simulink model "PositionComplementary4"  (Simulink 6.6)
settings: Solver=ode4  StartTime=0.0  StopTime=inf  FixedStep=SampleT  RelTol=1e-3
InitFcn:
  | clc
  | Taxi_Var_new
  | failures
  | insInit
  | piccolo_init
values from neighbouring files (symbols this model uses):
  A1 = 0    [Taxi_Var.m]    (also in Taxi_Var_new.m = 0.007)
  Apolar = 0.0899    [Taxi_Var.m]    (also in Taxi_Var_new.m = 0.057)
  CD0 = 0.0219    [Taxi_Var.m]    (also in Taxi_Var_new.m = 0.022)
  chord = S/span    (= 0.384036716878)    [Taxi_Var.m]    (also in Taxi_Var_new.m = 0.351341681574)
  CL0 = 0.1857    [Taxi_Var.m]    (also in Taxi_Var_new.m = 0.38)
  CLa = 4.6206    [Taxi_Var.m]    (also in Taxi_Var_new.m = 18.5)
  CLa_dot = 1.93    [Taxi_Var.m]    (also in Taxi_Var_new.m = 2.64)
  Clb = -0.0043    [Taxi_Var.m]    (also in Taxi_Var_new.m = -0.06)
  ClDa = 0.1695    [Taxi_Var.m]    (also in Taxi_Var_new.m)
  CLDe = 0.4032    [Taxi_Var.m]    (also in Taxi_Var_new.m = 0.24)
  CLDf = 0.047    [Taxi_Var.m]    (also in Taxi_Var_new.m = 0.4)
  ClDr = 0.0003    [Taxi_Var.m]    (also in Taxi_Var_new.m = 0.055)
  Clp = -0.4425    [Taxi_Var.m]    (also in Taxi_Var_new.m = -0.88)
  CLq = 8.7465    [Taxi_Var.m]    (also in Taxi_Var_new.m = 7.4)
  Clr = 0.0675    [Taxi_Var.m]    (also in Taxi_Var_new.m = 0.04)
  Cm0 = -0.0902    [Taxi_Var.m]    (also in Taxi_Var_new.m = 0.56)
  Cma = -1.3995    [Taxi_Var.m]    (also in Taxi_Var_new.m = -1.58)
  CmDe = -0.9493    [Taxi_Var.m]    (also in Taxi_Var_new.m = -41)
  CmDf = -.021    (= -0.021)    [Taxi_Var.m]    (also in Taxi_Var_new.m)
  Cmq = -10.8760    (= -10.876)    [Taxi_Var.m]    (also in Taxi_Var_new.m = -12)
  Cnb = 0.0281    [Taxi_Var.m]    (also in Taxi_Var_new.m = 0.73)
  CnDa = -0.0031    [Taxi_Var.m]    (also in Taxi_Var_new.m = -0.032)
  CnDr = -0.0882    [Taxi_Var.m]    (also in Taxi_Var_new.m = 0.19)
  Cnp = -0.0695    [Taxi_Var.m]    (also in Taxi_Var_new.m = -0.1)
  Cnr = -0.1045    [Taxi_Var.m]    (also in Taxi_Var_new.m = -0.23)
  CYb = -0.1999    [Taxi_Var.m]    (also in Taxi_Var_new.m = -0.98)
  CYDr = 0.0192    [Taxi_Var.m]    (also in Taxi_Var_new.m = 0.066)
  damax = 25*deg2rad    (= 0.436332312999)    [Taxi_Var.m]    (also in piccolo_init.m)
  damin = -25*deg2rad    (= -0.436332312999)    [Taxi_Var.m]    (also in piccolo_init.m)
  datrim = 0*deg2rad    (= 0)    [Taxi_Var.m]    (also in piccolo_init.m)
  demax = 15*deg2rad    (= 0.261799387799)    [Taxi_Var.m]    (also in piccolo_init.m)
  demin = -15*deg2rad    (= -0.261799387799)    [Taxi_Var.m]    (also in piccolo_init.m)
  detrim = -2.4137*deg2rad    (= -0.0421270121554)    [Taxi_Var.m]    (also in piccolo_init.m = -0.0523598775598)
  dfland = 30*deg2rad    (= 0.523598775598)    [Taxi_Var.m]    (also in piccolo_init.m)
  dfmax = 30*deg2rad    (= 0.523598775598)    [Taxi_Var.m]    (also in piccolo_init.m)
  dfmin = 0*deg2rad    (= 0)    [Taxi_Var.m]    (also in piccolo_init.m)
  drmax = 25*deg2rad    (= 0.436332312999)    [Taxi_Var.m]    (also in piccolo_init.m)
  drmin = -25*deg2rad    (= -0.436332312999)    [Taxi_Var.m]    (also in piccolo_init.m)
  drtrim = 0*deg2rad    (= 0)    [Taxi_Var.m]    (also in piccolo_init.m)
  dtmax = 1    [Taxi_Var.m]    (also in piccolo_init.m = 0.7)
  dtmin = 0    [Taxi_Var.m]    (also in piccolo_init.m = 0.25)
  dttrim = 0.0725    [Taxi_Var.m]    (also in piccolo_init.m = 0.35)
  Euler_0 = [0; 0; 45]'*pi/180    [Taxi_Var.m]    (also in Taxi_Var_new.m = [0 0 45]'*pi/180)
  IdxCmdOrbitRadius = 17    [piccolo_init.m]
  IdxCmdOrbitSense = 18    [piccolo_init.m]
  IdxCmdWp1Alt = 13    [piccolo_init.m]
  IdxCmdWp1Lat = 11    [piccolo_init.m]
  IdxCmdWp1Lon = 12    [piccolo_init.m]
  IdxCmdWp2Alt = 16    [piccolo_init.m]
  IdxCmdWp2Lat = 14    [piccolo_init.m]
  IdxCmdWp2Lon = 15    [piccolo_init.m]
  IdxEstimReserved1 = 4    [piccolo_init.m]
  IdxEstimWEast = 3    [piccolo_init.m]
  IdxEstimWNorth = 2    [piccolo_init.m]
  IdxGainsAltD = 10    [piccolo_init.m]
  IdxGainsAltI = 9    [piccolo_init.m]
  IdxGainsAltP = 8    [piccolo_init.m]
  IdxGainsPdynD = 4    [piccolo_init.m]
  IdxGainsPdynI = 3    [piccolo_init.m]
  IdxGainsPdynP = 2    [piccolo_init.m]
  IdxGainsPitchD = 7    [piccolo_init.m]
  IdxGainsPitchI = 6    [piccolo_init.m]
  IdxGainsPitchP = 5    [piccolo_init.m]
  IdxGainsRollD = 17    [piccolo_init.m]
  IdxGainsRollI = 16    [piccolo_init.m]
  IdxGainsRollP = 15    [piccolo_init.m]
  IdxGainsSlopeElevatorD = 25    [piccolo_init.m]
  IdxGainsSlopeElevatorP = 26    [piccolo_init.m]
  IdxGainsTrackConv = 24    [piccolo_init.m]
  IdxGainsTrackD = 23    [piccolo_init.m]
  IdxGainsTrackI = 22    [piccolo_init.m]
  IdxGainsTrackP = 21    [piccolo_init.m]
  IdxGainsTurnD = 14    [piccolo_init.m]
  IdxGainsTurnI = 13    [piccolo_init.m]
  IdxGainsTurnP = 12    [piccolo_init.m]
  IdxGainsYawD = 20    [piccolo_init.m]
  IdxGainsYawI = 19    [piccolo_init.m]
  IdxGainsYawP = 18    [piccolo_init.m]
  IdxLimitsAileronMax = 11    [piccolo_init.m]
  IdxLimitsAileronMin = 10    [piccolo_init.m]
  IdxLimitsBankMax = 9    [piccolo_init.m]
  IdxLimitsBankMin = 8    [piccolo_init.m]
  IdxLimitsElevatorMax = 13    [piccolo_init.m]
  IdxLimitsElevatorMin = 12    [piccolo_init.m]
  IdxLimitsFlapMax = 19    [piccolo_init.m]
  IdxLimitsFlapMin = 18    [piccolo_init.m]
  IdxLimitsPdynMax = 3    [piccolo_init.m]
  IdxLimitsPdynMin = 2    [piccolo_init.m]
  IdxLimitsRudderMax = 15    [piccolo_init.m]
  IdxLimitsRudderMin = 14    [piccolo_init.m]
  IdxLimitsThrottleMax = 17    [piccolo_init.m]
  IdxLimitsThrottleMin = 16    [piccolo_init.m]
  IdxSensorsAlt = 5    [piccolo_init.m]
  IdxSensorsLat = 3    [piccolo_init.m]
  IdxSensorsLon = 4    [piccolo_init.m]
  IdxSensorsVDown = 8    [piccolo_init.m]
  IdxSensorsVEast = 7    [piccolo_init.m]
  IdxSensorsVNorth = 6    [piccolo_init.m]
  IdxStatesGlobal = 2    [piccolo_init.m]
  IdxStatesManual = 16    [piccolo_init.m]
  IdxStatesMode = 15    [piccolo_init.m]
  ISA_g = 9.815    [Taxi_Var.m]    (also in Taxi_Var_new.m)
  ISA_hmax = 2000    [Taxi_Var.m]    (also in Taxi_Var_new.m)
  ISA_lapse = .0065    (= 0.0065)    [Taxi_Var.m]    (also in Taxi_Var_new.m)
  ISA_P0 = 101325    [Taxi_Var.m]    (also in Taxi_Var_new.m)
  ISA_R = 287    [Taxi_Var.m]    (also in Taxi_Var_new.m)
  ISA_rho0 = 1.225    [Taxi_Var.m]    (also in Taxi_Var_new.m)
  ISA_T0 = 289    [Taxi_Var.m]    (also in Taxi_Var_new.m)
  Ixx = 3.689084    [Taxi_Var.m]    (also in Taxi_Var_new.m = 3.8)
  Iyy = 7.43789    [Taxi_Var.m]    (also in Taxi_Var_new.m = 9.58)
  Izz = 10.22202    [Taxi_Var.m]    (also in Taxi_Var_new.m = 9.68)
  mass = 22.5    [Taxi_Var.m]    (also in Taxi_Var_new.m = 8.16466266)
  MinThK = 0.075    [Taxi_Var.m]    (also in Taxi_Var_new.m = 0.077)
  Pos_0 = [0; 0; 1000]'    [Taxi_Var.m]    (also in Taxi_Var_new.m = [0 0 500]')
  PQR_0 = [0; 0; 0]'    [Taxi_Var.m]    (also in Taxi_Var_new.m = [ 0 0 0]'*pi/180)
  SampleT = 0.005    [failures.m]
  span = 2.3368    [Taxi_Var.m]    (also in Taxi_Var_new.m = 2.795)
  TFact = 0.4    [Taxi_Var.m]    (also in Taxi_Var_new.m)
  ThK = 2.18    [Taxi_Var.m]    (also in Taxi_Var_new.m = 2.17)
  tsamp = APtsamp    (= 0.05)    [piccolo_init.m]
  ... (+1 more)
undefined symbols (not defined in the file or in its folder): clock, DiscIntNeverNeededParam, Earth, gaind, polesd, WGS84, zerosd
libraries: piccolo_library x60, simulink x55, aerolibconvert2 x18, aerolibasang x5, dspsigops x5, aerolibtransform2 x2, aerolibatmos2 x2, aerolibnav x2, aerolibguid x1, aerolibutil x1, dspmtrx3 x1
(part 2 of 7)

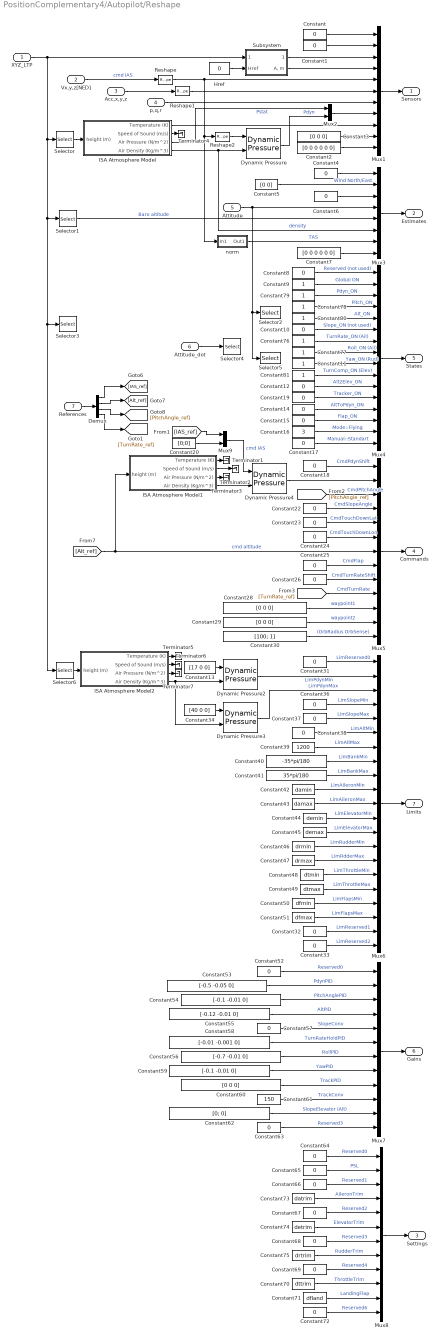
== system PositionComplementary4/Autopilot/Reshape ==
  XYZ_LTP : Inport  OutDataType=fixdt(1,16,0)  OutScaling=[]
  Vx,y,z[NED] : Inport  Port=2  OutDataType=fixdt(1,16,0)  OutScaling=[]
  Acc,x,y,z : Inport  Port=3  OutDataType=fixdt(1,16,0)  OutScaling=[]
  p,q,r : Inport  Port=4  OutDataType=fixdt(1,16,0)  OutScaling=[]
  Attitude : Inport  Port=5  OutDataType=fixdt(1,16,0)  OutScaling=[]
  Attitude_dot : Inport  Port=6  OutDataType=fixdt(1,16,0)  OutScaling=[]
  References : Inport  Port=7  OutDataType=fixdt(1,16,0)  OutScaling=[]
  Constant{,1,4,6,8,10,12,14..15,17..19,22..26,31..33,36..38,52,57,63..69,72} (33 alike) : Constant  Value=0
  Constant{9,11,76..81} (8 alike) : Constant
  Constant13 : Constant  Value=[17 0 0]
  Constant16 : Constant  Value=3
  Constant2 : Constant  Value=[0 0 0 0 0 0]
  Constant20 : Constant  Value=[0;0]
  Constant{3,28..29,60} (4 alike) : Constant  Value=[0 0 0]
  Constant30 : Constant  Value=[100; 1]
  Constant34 : Constant  Value=[40 0 0]
  Constant39 : Constant  Value=1200
  Constant40 : Constant  Value=-35*pi/180
  Constant41 : Constant  Value=35*pi/180
  Constant42 : Constant  Value=damin
  Constant43 : Constant  Value=damax
  Constant44 : Constant  Value=demin
  Constant45 : Constant  Value=demax
  Constant46 : Constant  Value=drmin
  Constant47 : Constant  Value=drmax
  Constant48 : Constant  Value=dtmin
  Constant49 : Constant  Value=dtmax
  Constant5 : Constant  Value=[0 0]
  Constant50 : Constant  Value=dfmin
  Constant51 : Constant  Value=dfmax
  Constant53 : Constant  Value=[-0.5 -0.05 0]
  Constant54 : Constant  Value=[-0.1 -0.01 0]
  Constant55 : Constant  Value=[-0.12 -0.01 0]
  Constant56 : Constant  Value=[-0.7 -0.01 0]
  Constant58 : Constant  Value=[-0.01 -0.001 0]
  Constant59 : Constant  Value=[-0.1 -0.01 0]
  Constant61 : Constant  Value=150
  Constant62 : Constant  Value=[0; 0]
  Constant7 : Constant  Value=[0 0 0 0 0 0]
  Constant70 : Constant  Value=dttrim
  Constant71 : Constant  Value=dfland
  Constant73 : Constant  Value=datrim
  Constant74 : Constant  Value=detrim
  Constant75 : Constant  Value=drtrim
  Demux : Demux
  Dynamic Pressure{,2..4} (4 alike) : aerolibasang/Dynamic Pressure  SystemSampleTime=-1
  Href : Constant  Value=0
  ISA Atmosphere Model : Subsystem  mask(International Standart Atmosphere){L=ISA_lapse, h_lim=ISA_hmax, R=ISA_R, g=ISA_g, rh0=ISA_rho0, P0=ISA_P0, T0=ISA_T0}
      mask prompts: L "Lapse rate"; h_lim "Upper altitude limit, (m)"; R "Universal gas constant R"; g "Garvity constant, (m/c^2)"; rh0 "Sea level density, (kg/m^3)"; P0 "Sea level pressure, (N/m^2)"; T0 "Sea level temperature, (K)"
  ISA Atmosphere Model1 : Subsystem  mask(International Standart Atmosphere){L=ISA_lapse, h_lim=ISA_hmax, R=ISA_R, g=ISA_g, rh0=ISA_rho0, P0=ISA_P0, T0=ISA_T0}
      mask prompts: L "Lapse rate"; h_lim "Upper altitude limit, (m)"; R "Universal gas constant R"; g "Garvity constant, (m/c^2)"; rh0 "Sea level density, (kg/m^3)"; P0 "Sea level pressure, (N/m^2)"; T0 "Sea level temperature, (K)"
  ISA Atmosphere Model2 : Subsystem  mask(International Standart Atmosphere){L=ISA_lapse, h_lim=ISA_hmax, R=ISA_R, g=ISA_g, rh0=ISA_rho0, P0=ISA_P0, T0=ISA_T0}
      mask prompts: L "Lapse rate"; h_lim "Upper altitude limit, (m)"; R "Universal gas constant R"; g "Garvity constant, (m/c^2)"; rh0 "Sea level density, (kg/m^3)"; P0 "Sea level pressure, (N/m^2)"; T0 "Sea level temperature, (K)"
  Mux1 : Mux  Inputs=11
  Mux2 : Mux  Inputs=2
  Mux3 : Mux  Inputs=8
  Mux4 : Mux  Inputs=16
  Mux5 : Mux  Inputs=13
  Mux6 : Mux  Inputs=21
  Mux7 : Mux  Inputs=12
  Mux8 : Mux  Inputs=12
  Mux9 : Mux  Inputs=2
  Reshape : Reshape
  Reshape1 : Reshape
  Reshape2 : Reshape
  Selector{,1,3..4,6} (5 alike) : Selector  IndexOptions=Index vector (dialog)  Indices=3  OutputSizes=[(-2)]  InputPortWidth=3
  Selector2 : Selector  IndexOptions=Index vector (dialog)  Indices=2  OutputSizes=[(-2)]  InputPortWidth=3
  Selector5 : Selector  IndexOptions=Index vector (dialog)  Indices=[1 3]  OutputSizes=[(-2)]  InputPortWidth=3
  Subsystem : Subsystem
  Terminator{1..7} (7 alike) : Terminator
  norm : Subsystem
  Sensors : Outport  OutDataType=fixdt(1,16,0)  OutScaling=[]
  Estimates : Outport  Port=2  OutDataType=fixdt(1,16,0)  OutScaling=[]
  Settings : Outport  Port=3  OutDataType=fixdt(1,16,0)  OutScaling=[]
  Commands : Outport  Port=4  OutDataType=fixdt(1,16,0)  OutScaling=[]
  States : Outport  Port=5  OutDataType=fixdt(1,16,0)  OutScaling=[]
  Gains : Outport  Port=6  OutDataType=fixdt(1,16,0)  OutScaling=[]
  Limits : Outport  Port=7  OutDataType=fixdt(1,16,0)  OutScaling=[]
  wires:
  Constant/1 -> Mux1/1
  Constant1/1 -> Mux1/2
  Subsystem/1("LL, deg") -> Mux1/3
  Subsystem/2("A, m") -> Mux1/4
  XYZ_LTP/1 -> Subsystem/1("XYZ, ltp"), Selector/1, Selector1/1, Selector3/1, Selector6/1
  Vx,y,z[NED]/1 -> Reshape/1  "cmd IAS"
  Mux1/1 -> Sensors/1
  Acc,x,y,z/1 -> Reshape1/1
  p,q,r/1 -> Mux1/7
  Constant3/1 -> Mux1/10
  Constant2/1 -> Mux1/11
  ISA Atmosphere Model/4(Air Density (Kg/m^3)) -> Dynamic Pressure/2, Mux3/6  "density"
  ISA Atmosphere Model/1(Temperature (K)) -> Mux1/9
  Mux2/1 -> Mux1/8
  ISA Atmosphere Model/3("Air Pressure (N/m^2) ") -> Mux2/1  "Pstat"
  ISA Atmosphere Model/2("Speed of Sound (m/s) ") -> Terminator4/1
  Dynamic Pressure/1 -> Mux2/2  "Pdyn"
  Selector/1 -> ISA Atmosphere Model/1(height (m))
  Reshape/1 -> Mux1/5, Reshape2/1, norm/1(In1)
  Reshape1/1 -> Mux1/6
  Reshape2/1 -> Dynamic Pressure/1
  Href/1 -> Subsystem/2(Href)
  Mux3/1 -> Estimates/1
  Constant4/1 -> Mux3/1
  Constant5/1 -> Mux3/2  "Wind North/East"
  Constant6/1 -> Mux3/3
  Attitude/1 -> Selector2/1, Selector5/1, Mux3/4
  Selector1/1 -> Mux3/5  "Baro altitude"
  norm/1(Out1) -> Mux3/7  "TAS"
  Constant7/1 -> Mux3/8
  Mux4/1 -> States/1
  Constant8/1 -> Mux4/1  "Reserved (not used)"
  Constant9/1 -> Mux4/2  "Global ON"
  Constant10/1 -> Mux4/6  "Slope_ON (not used)"
  Attitude_dot/1 -> Selector4/1
  Constant11/1 -> Mux4/9  "Yaw_ON (Rud)"
  Mux5/1 -> Commands/1
  Constant18/1 -> Mux5/1  "CmdPdynShift"
  ISA Atmosphere Model1/1(Temperature (K)) -> Terminator1/1
  ISA Atmosphere Model1/2("Speed of Sound (m/s) ") -> Terminator2/1
  ISA Atmosphere Model1/3("Air Pressure (N/m^2) ") -> Terminator3/1
  ISA Atmosphere Model1/4(Air Density (Kg/m^3)) -> Dynamic Pressure4/2
  Dynamic Pressure4/1 -> Mux5/2
  Mux9/1 -> Dynamic Pressure4/1  "cmd IAS"
  [Alt_ref] -> ISA Atmosphere Model1/1(height (m)), Mux5/7  "cmd altitude"
  [PitchAngle_ref] -> Mux5/3  "CmdPitchAngle"
  Constant22/1 -> Mux5/4  "CmdSlopeAngle"
  Constant24/1 -> Mux5/6  "CmdTouchDownLon"
  Constant23/1 -> Mux5/5  "CmdTouchDownLat"
  Constant25/1 -> Mux5/8  "CmdFlap"
  Constant26/1 -> Mux5/9  "CmdTurnRateShift"
  [TurnRate_ref] -> Mux5/10  "CmdTurnRate"
  Constant28/1 -> Mux5/11  "waypoint1"
  Constant29/1 -> Mux5/12  "waypoint2"
  Constant30/1 -> Mux5/13  "(OrbRadius OrbSense)"
  Mux6/1 -> Limits/1
  Constant31/1 -> Mux6/1  "LimReserved0"
  Constant33/1 -> Mux6/21  "LimReserved2"
  Constant32/1 -> Mux6/20  "LimReserved1"
  ISA Atmosphere Model2/1(Temperature (K)) -> Terminator5/1
  ISA Atmosphere Model2/2("Speed of Sound (m/s) ") -> Terminator6/1
  ISA Atmosphere Model2/3("Air Pressure (N/m^2) ") -> Terminator7/1
  ISA Atmosphere Model2/4(Air Density (Kg/m^3)) -> Dynamic Pressure2/2, Dynamic Pressure3/2
  Constant13/1 -> Dynamic Pressure2/1
  Constant34/1 -> Dynamic Pressure3/1
  Selector6/1 -> ISA Atmosphere Model2/1(height (m))
  Dynamic Pressure2/1 -> Mux6/2  "LimPdynMin"
  Dynamic Pressure3/1 -> Mux6/3  "LimPdynMax"
  Constant36/1 -> Mux6/4  "LimSlopeMin"
  Constant37/1 -> Mux6/5  "LimSlopeMax"
  Constant38/1 -> Mux6/6  "LimAltMin"
  Constant39/1 -> Mux6/7  "LimAltMax"
  Constant40/1 -> Mux6/8  "LimBankMin"
  Constant41/1 -> Mux6/9  "LimBankMax"
  Constant42/1 -> Mux6/10  "LimAileronMin"
  Constant43/1 -> Mux6/11  "LimAileronMax"
  Constant44/1 -> Mux6/12  "LimElevatorMin"
  Constant45/1 -> Mux6/13  "LimElevatorMax"
  Constant46/1 -> Mux6/14  "LimRudderMin"
  Constant47/1 -> Mux6/15  "LimRdderMax"
  Constant48/1 -> Mux6/16  "LimThrottleMin"
  Constant49/1 -> Mux6/17  "LimThrottleMax"
  Constant50/1 -> Mux6/18  "LimFlapsMin"
  Constant51/1 -> Mux6/19  "LimFlapsMax"
  Mux7/1 -> Gains/1
  Constant52/1 -> Mux7/1  "Reserved0"
  Constant53/1 -> Mux7/2  "PdynPID"
  Constant54/1 -> Mux7/3  "PitchAnglePID"
  Constant55/1 -> Mux7/4  "AltPID"
  Constant58/1 -> Mux7/6  "TurnRateHoldPID"
  Constant57/1 -> Mux7/5  "SlopeConv"
  Constant56/1 -> Mux7/7  "RollPID"
  Constant59/1 -> Mux7/8  "YawPID"
  Constant60/1 -> Mux7/9  "TrackPID"
  Constant61/1 -> Mux7/10  "TrackConv"
  Constant62/1 -> Mux7/11  "SlopeElevator (Alt)"
  Constant63/1 -> Mux7/12  "Reserved3"
  Mux8/1 -> Settings/1
  Constant64/1 -> Mux8/1  "Reserved0"
  Constant65/1 -> Mux8/2  "PSL"
  Constant66/1 -> Mux8/3  "Reserved1"
  Constant67/1 -> Mux8/5  "Reserved2"
  Constant68/1 -> Mux8/7  "Reserved3"
  Constant69/1 -> Mux8/9  "Reserved4"
  Constant70/1 -> Mux8/10  "ThrottleTrim"
  Constant71/1 -> Mux8/11  "LandingFlap"
  Constant72/1 -> Mux8/12  "Reserved6"
  Constant73/1 -> Mux8/4  "AileronTrim"
  Constant74/1 -> Mux8/6  "ElevatorTrim"
  Constant75/1 -> Mux8/8  "RudderTrim"
  Constant76/1 -> Mux4/7  "TurnRate_ON (Ail)"
  Constant77/1 -> Mux4/8  "Roll_ON (Ail)"
  Constant78/1 -> Mux4/4  "Pitch_ON"
  Constant79/1 -> Mux4/3  "Pdyn_ON"
  Constant80/1 -> Mux4/5  "Alt_ON"
  Constant81/1 -> Mux4/10  "TurnComp_ON (Elev)"
  Constant12/1 -> Mux4/11  "Alt2Elev_ON"
  Constant19/1 -> Mux4/12  "Tracker_ON"
  Constant14/1 -> Mux4/13  "AltToPdyn_ON"
  Constant15/1 -> Mux4/14  "Flap_ON"
  Constant16/1 -> Mux4/15  "Mode::Flying"
  Constant17/1 -> Mux4/16  "Manual::Standart"
  References/1 -> Demux/1
  Demux/1 -> [IAS_ref]
  Demux/2 -> [Alt_ref]
  Demux/3 -> [PitchAngle_ref]
  Demux/4 -> [TurnRate_ref]
  Constant20/1 -> Mux9/2
  [IAS_ref] -> Mux9/1

== system PositionComplementary4/GPS Update/Detect Change ==
  Data : Inport
  Abs1 : Abs  SampleTime=T
  Difference1 : simulink/Discrete/Difference  SystemSampleTime=-1  ICPrevInput=0.0  OutDataType=sfix(16)  OutScaling=2^-10  DoSatur=off
  Saturation1 : Saturate  UpperLimit=1  LowerLimit=0  SampleTime=T
  change? : Outport
  wires:
  Difference1/1 -> Abs1/1
  Abs1/1 -> Saturation1/1
  Data/1 -> Difference1/1
  Saturation1/1 -> change?/1

== system PositionComplementary4/GPS Update/Detect Change1 ==
  Data : Inport
  Abs1 : Abs  SampleTime=T
  Difference1 : simulink/Discrete/Difference  SystemSampleTime=-1  ICPrevInput=0.0  OutDataType=sfix(16)  OutScaling=2^-10  DoSatur=off
  Saturation1 : Saturate  UpperLimit=1  LowerLimit=0  SampleTime=T
  change? : Outport
  wires:
  Saturation1/1 -> change?/1
  Data/1 -> Difference1/1
  Abs1/1 -> Saturation1/1
  Difference1/1 -> Abs1/1

== system PositionComplementary4/GPS Update/Detect Change2 ==
  Data : Inport
  Abs1 : Abs  SampleTime=T
  Difference1 : simulink/Discrete/Difference  SystemSampleTime=-1  ICPrevInput=0.0  OutDataType=sfix(16)  OutScaling=2^-10  DoSatur=off
  Saturation1 : Saturate  UpperLimit=1  LowerLimit=0  SampleTime=T
  change? : Outport
  wires:
  Difference1/1 -> Abs1/1
  Abs1/1 -> Saturation1/1
  Data/1 -> Difference1/1
  Saturation1/1 -> change?/1

== system PositionComplementary4/Get GPS in LTP/Geod2LTP2 ==
  "Height, Lat, Lon Initials from GPS" : Inport
  "Lat, deg(GPS)" : Inport  Port=2
  "Lon, deg(GPS)" : Inport  Port=3
  Hight,m(GPS) : Inport  Port=4
  Demux : Demux  Outputs=3
  ECEF2LTP (UEN) : Subsystem
      mask Display: plot(0,0,100,100,[45,40,35,40,40],[85,95,85,95,40],[85,95,85,95,40],[35,40,45,40,40],[60,40,10,20,10,14],[70,40,10,13,10,20],[56,45],[70,70],[60,60],[50,60],[60,60],[30,40],[50,60],[20,20],[30,40],[20,20],[45,55],[35,25],[75,65],[35,25])
  Geod2ECEF : Subsystem  mask{Re=6378137, Rp=6356752.3142}
      mask prompts: Re "Enter equatorial radius, m"; Rp "Enter polar radius,m"
  Geod2ECEF1 : Subsystem  mask{Re=6378137, Rp=6356752.3142}
      mask prompts: Re "Enter equatorial radius, m"; Rp "Enter polar radius,m"
  Mux : Mux  Inputs=3
  Mux1 : Mux  Inputs=2
  Mux2 : Mux  Inputs=3
  Reshape : Reshape  OutputDimensionality=Column vector (2-D)
  Sum1 : Sum  Inputs=|+-  SaturateOnIntegerOverflow=on
  UEN 2 NEU : Gain  Gain=[0 0 1;0 1 0;1 0 0]  Multiplication=Matrix(K*u)  SaturateOnIntegerOverflow=on
  "NEU, m" : Outport
  wires:
  UEN 2 NEU/1 -> "NEU, m"/1
  Geod2ECEF/3("Ze, m ") -> Mux/3
  Geod2ECEF/1("Xe, m ") -> Mux/1
  Geod2ECEF/2("Ye, m ") -> Mux/2
  "Lat, deg(GPS)"/1 -> Geod2ECEF/2("lat, deg")
  "Lon, deg(GPS)"/1 -> Geod2ECEF/3(lon,deg)
  Mux1/1 -> ECEF2LTP (UEN)/2("Long, Lat")
  Geod2ECEF1/3("Ze, m ") -> Mux2/3
  Geod2ECEF1/1("Xe, m ") -> Mux2/1
  Geod2ECEF1/2("Ye, m ") -> Mux2/2
  Mux2/1 -> Sum1/2  "R_in"
  Demux/1 -> Geod2ECEF1/1("height, m")
  Demux/2 -> Mux1/2, Geod2ECEF1/2("lat, deg")
  Demux/3 -> Mux1/1, Geod2ECEF1/3(lon,deg)
  ECEF2LTP (UEN)/1(Out) -> Reshape/1  "Moving Side"
  Hight,m(GPS)/1 -> Geod2ECEF/1("height, m")
  "Height, Lat, Lon Initials from GPS"/1 -> Demux/1
  Mux/1 -> Sum1/1  "r_mov"
  Sum1/1 -> ECEF2LTP (UEN)/1(ECEF coordinates)
  Reshape/1 -> UEN 2 NEU/1

== system PositionComplementary4/Get GPS in LTP/Sim Latency ==
  Fast Data : Inport
  Data Type Conversion : DataTypeConversion  OutDataTypeMode=double
  Pulse Generator : DiscretePulseGenerator  PulseType=Time based  PulseWidth=50
  Rate Transition2 : RateTransition  OutPortSampleTime=SampleT
  Sample and Hold : dspsigops/Sample and Hold  SystemSampleTime=-1  trig=Either edge  initCond=0  latchinput=off
  1Hz Data : Outport
  wires:
  Data Type Conversion/1 -> Rate Transition2/1
  Sample and Hold/1 -> 1Hz Data/1
  Fast Data/1 -> Sample and Hold/1
  Rate Transition2/1 -> Sample and Hold/Trigger
  Pulse Generator/1 -> Data Type Conversion/1

== system PositionComplementary4/Get GPS in LTP/Sim Latency1 ==
  Fast Data : Inport
  Data Type Conversion : DataTypeConversion  OutDataTypeMode=double
  Pulse Generator : DiscretePulseGenerator  PulseType=Time based  PulseWidth=50
  Rate Transition2 : RateTransition  OutPortSampleTime=SampleT
  Sample and Hold : dspsigops/Sample and Hold  SystemSampleTime=-1  trig=Either edge  initCond=0  latchinput=off
  1Hz Data : Outport
  wires:
  Pulse Generator/1 -> Data Type Conversion/1
  Rate Transition2/1 -> Sample and Hold/Trigger
  Fast Data/1 -> Sample and Hold/1
  Sample and Hold/1 -> 1Hz Data/1
  Data Type Conversion/1 -> Rate Transition2/1

== system PositionComplementary4/Get GPS in LTP/Sim Latency2 ==
  Fast Data : Inport
  Data Type Conversion : DataTypeConversion  OutDataTypeMode=double
  Pulse Generator : DiscretePulseGenerator  PulseType=Time based  PulseWidth=50
  Rate Transition2 : RateTransition  OutPortSampleTime=SampleT
  Sample and Hold : dspsigops/Sample and Hold  SystemSampleTime=-1  trig=Either edge  initCond=0  latchinput=off
  1Hz Data : Outport
  wires:
  Data Type Conversion/1 -> Rate Transition2/1
  Sample and Hold/1 -> 1Hz Data/1
  Fast Data/1 -> Sample and Hold/1
  Rate Transition2/1 -> Sample and Hold/Trigger
  Pulse Generator/1 -> Data Type Conversion/1

== system PositionComplementary4/Get GPS in LTP/Sim Latency3 ==
  Fast Data : Inport
  Data Type Conversion : DataTypeConversion  OutDataTypeMode=double
  Pulse Generator : DiscretePulseGenerator  PulseType=Time based  PulseWidth=50
  Rate Transition2 : RateTransition  OutPortSampleTime=SampleT
  Sample and Hold : dspsigops/Sample and Hold  SystemSampleTime=-1  trig=Either edge  initCond=0  latchinput=off
  1Hz Data : Outport
  wires:
  Pulse Generator/1 -> Data Type Conversion/1
  Rate Transition2/1 -> Sample and Hold/Trigger
  Fast Data/1 -> Sample and Hold/1
  Sample and Hold/1 -> 1Hz Data/1
  Data Type Conversion/1 -> Rate Transition2/1

== system PositionComplementary4/Get GPS in LTP/Sim Latency4 ==
  Fast Data : Inport
  Data Type Conversion : DataTypeConversion  OutDataTypeMode=double
  Pulse Generator : DiscretePulseGenerator  PulseType=Time based  PulseWidth=50
  Rate Transition2 : RateTransition  OutPortSampleTime=SampleT
  Sample and Hold : dspsigops/Sample and Hold  SystemSampleTime=-1  trig=Either edge  initCond=0  latchinput=off
  1Hz Data : Outport
  wires:
  Data Type Conversion/1 -> Rate Transition2/1
  Sample and Hold/1 -> 1Hz Data/1
  Fast Data/1 -> Sample and Hold/1
  Rate Transition2/1 -> Sample and Hold/Trigger
  Pulse Generator/1 -> Data Type Conversion/1

== system PositionComplementary4/Plant Model/Plant ==
  de : Inport
  da : Inport  Port=2
  dr : Inport  Port=3
  dt : Inport  Port=4
  df : Inport  Port=5
  6-DOF EOM : Subsystem
  Engine Model : Subsystem
  Forces and Moments : Subsystem
  Get GPS : Subsystem
  ISA Atmosphere & Winds : Subsystem  Orientation=left
  Mux : Mux  Inputs=2
  Scope : Scope
      settings: YMin=0  YMax=5250
  Sum : Sum  Inputs=++|  SaturateOnIntegerOverflow=on
  Wrap Around PSI1 : Subsystem
  GPS Month : Outport
  GPS Day : Outport  Port=2
  GPS Year : Outport  Port=3
  GPS Hr : Outport  Port=4
  GPS Min : Outport  Port=5
  GPS Sec : Outport  Port=6
  GPS Frac Sec : Outport  Port=7
  GPS Lat (rad) : Outport  Port=8
  GPS Long (rad) : Outport  Port=9
  GPS H (m) : Outport  Port=10
  PQR : Outport  Port=11
  Ab : Outport  Port=12
  Dynamic : Outport  Port=13
  Static : Outport  Orientation=left  Port=14
  Euler : Outport  Port=15
  Vmag : Outport  Port=16
  RPM : Outport  Port=17
  Vned : Outport  Port=18
  aoa/betta,deg : Outport  Port=19
  Ab meas : Outport  Port=20
  Vb : Outport  Port=21
  Euler_dot : Outport  Port=22
  wires:
  Get GPS/1(GPS Month) -> GPS Month/1
  Get GPS/2(GPS Day) -> GPS Day/1
  Get GPS/3(GPS Year) -> GPS Year/1
  Get GPS/4(GPS Hr) -> GPS Hr/1
  Get GPS/5(GPS Min) -> GPS Min/1
  Get GPS/6(GPS Sec) -> GPS Sec/1
  Get GPS/7(GPS Frac Sec) -> GPS Frac Sec/1
  Get GPS/8(GPS Lat (rad)) -> GPS Lat (rad)/1
  Get GPS/9(GPS Long (rad)) -> GPS Long (rad)/1
  Get GPS/10(GPS H (m)) -> GPS H (m)/1
  6-DOF EOM/8(Ab meas) -> Ab meas/1
  Mux/1 -> 6-DOF EOM/1("[F,M]")
  6-DOF EOM/5(Euler_dot) -> Euler_dot/1
  6-DOF EOM/6(Vb) -> Vb/1
  Engine Model/1(RPM) -> RPM/1
  Engine Model/2(Thrust) -> Sum/1
  Forces and Moments/6(q) -> Dynamic/1
  ISA Atmosphere & Winds/3(AirPressure (Pa)) -> Static/1
  Forces and Moments/1(Airspeed) -> Engine Model/2(Vmag), Vmag/1
  ISA Atmosphere & Winds/2(Wind) -> Forces and Moments/1(Wind e)
  ISA Atmosphere & Winds/1(Rho) -> Forces and Moments/2(Rho)
  Forces and Moments/3(Moments) -> Mux/2
  Forces and Moments/2(Forces) -> Sum/2
  Sum/1 -> Mux/1
  Forces and Moments/4(Vb Corr) -> 6-DOF EOM/2(Vb Corr)
  6-DOF EOM/1(X,Y,Z (LTP)) -> ISA Atmosphere & Winds/1("X, Y, Z"), Get GPS/1(XYZ (NEU)), Scope/1  "position"
  6-DOF EOM/2("Vx, Vy, Vz") -> Vned/1, Forces and Moments/7("Vx, Vy, Vz ")  "velocity"
  6-DOF EOM/3(Euler) -> Forces and Moments/8(Euler), Wrap Around PSI1/1(Euler)  "Euler angles"
  6-DOF EOM/4("p, q, r") -> PQR/1, Forces and Moments/9(p,q,r)  "rates"
  6-DOF EOM/7(Ab) -> Ab/1
  Forces and Moments/5("aoa/betta, deg") -> aoa/betta,deg/1
  dt/1 -> Engine Model/1(dt)
  de/1 -> Forces and Moments/3("de, deg")
  da/1 -> Forces and Moments/4(da,deg)
  dr/1 -> Forces and Moments/5("dr, deg")
  df/1 -> Forces and Moments/6("df, deg")
  Wrap Around PSI1/1(Euler-Wrapped) -> Euler/1

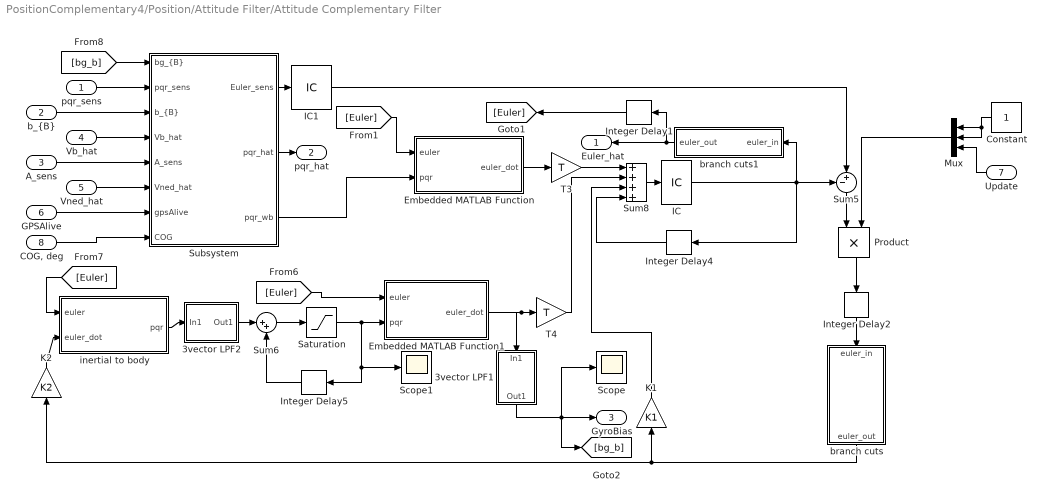
== system PositionComplementary4/Position/Attitude Filter/Attitude Complementary Filter ==
  pqr_sens : Inport
  "b_{B}" : Inport  Port=2
  A_sens : Inport  Port=3
  Vb_hat : Inport  Port=4
  Vned_hat : Inport  Port=5
  GPSAlive : Inport  Port=6
  Update : Inport  Orientation=left  Port=7
  "COG, deg" : Inport  Port=8
  3vector LPF1 : Subsystem  Orientation=down  mask{flpf=15, T=T}
      mask prompts: flpf "Low Pass Frequency (in S domain)"; T "Sample time"
      mask Display: droots([],-flpf,flpf)
  3vector LPF2 : Subsystem  mask{flpf=flpf, T=T}
      mask prompts: flpf "Low Pass Frequency (in S domain)"; T "Sample time"
      mask Display: droots([],-flpf,flpf)
  Constant : Constant  Orientation=left
  Embedded MATLAB Function : Stateflow chart
  Embedded MATLAB Function1 : Stateflow chart
  IC : InitialCondition  Value=P0  SampleTime=T
  IC1 : InitialCondition  Value=P0  SampleTime=T
  Integer Delay1 : simulink/Discrete/Integer Delay  Orientation=left  vinit=0.0  samptime=-1  NumDelays=1
  Integer Delay2 : simulink/Discrete/Integer Delay  Orientation=down  vinit=0.0  samptime=-1  NumDelays=1
  Integer Delay4 : simulink/Discrete/Integer Delay  Orientation=left  vinit=0.0  samptime=-1  NumDelays=1
  Integer Delay5 : simulink/Discrete/Integer Delay  Orientation=left  vinit=0.0  samptime=-1  NumDelays=1
  K1 : Gain  Orientation=up  Gain=K1
  K2 : Gain  Orientation=up  Gain=K2
  Mux : Mux  Orientation=left  Inputs=3
  Product : Product  Orientation=down  RndMeth=Zero
  Saturation : Saturate  UpperLimit=1.5  LowerLimit=-1.5
  Scope : Scope
      settings: TimeRange=60  YMin=-0.07116438310879042  YMax=0.01417979172834782  SaveName=ScopeData13
  Scope1 : Scope
      settings: TimeRange=60  YMin=-0.07116438310879042  YMax=0.01417979172834782  SaveName=ScopeData30
  Subsystem : Subsystem
  Sum5 : Sum  Orientation=down  Inputs=-+|
  Sum6 : Sum  Inputs=|++
  Sum8 : Sum  Inputs=4
  T3 : Gain  Gain=T  SampleTime=T
  T4 : Gain  Gain=T  SampleTime=T
  branch cuts : Stateflow chart  Orientation=down
  branch cuts1 : Stateflow chart  Orientation=left
  inertial to body : Stateflow chart
  Euler_hat : Outport  Orientation=left
  pqr_hat : Outport  Port=2
  GyroBias : Outport  Port=3
  wires:
  Embedded MATLAB Function/1(euler_dot) -> T3/1
  Subsystem/1(Euler_sens) -> IC1/1
  T3/1 -> Sum8/1
  Sum8/1 -> IC/1
  Integer Delay4/1 -> Sum8/4
  K1/1 -> Sum8/3
  inertial to body/1(pqr) -> 3vector LPF2/1(In1)
  Sum6/1 -> Saturation/1
  [Euler] -> Embedded MATLAB Function1/1(euler)
  [Euler] -> inertial to body/1(euler)
  Embedded MATLAB Function1/1(euler_dot) -> T4/1, 3vector LPF1/1(In1)
  T4/1 -> Sum8/2
  Integer Delay5/1 -> Sum6/2
  K2/1 -> inertial to body/2(euler_dot)
  [bg_b] -> Subsystem/1("bg_{B}")
  pqr_sens/1 -> Subsystem/2(pqr_sens)
  "b_{B}"/1 -> Subsystem/3("b_{B}")
  Vb_hat/1 -> Subsystem/4(Vb_hat)
  A_sens/1 -> Subsystem/5(A_sens)
  Vned_hat/1 -> Subsystem/6(Vned_hat)
  IC/1 -> Integer Delay4/1, Sum5/1, branch cuts1/1(euler_in)
  IC1/1 -> Sum5/2
  Integer Delay1/1 -> [Euler]
  [Euler] -> Embedded MATLAB Function/1(euler)
  Integer Delay2/1 -> branch cuts/1(euler_in)
  Subsystem/3(pqr_wb) -> Embedded MATLAB Function/2(pqr)
  Subsystem/2(pqr_hat) -> pqr_hat/1
  branch cuts/1(euler_out) -> K2/1, K1/1
  branch cuts1/1(euler_out) -> Euler_hat/1, Integer Delay1/1
  GPSAlive/1 -> Subsystem/7(gpsAlive)
  Product/1 -> Integer Delay2/1
  Sum5/1 -> Product/1
  "COG, deg"/1 -> Subsystem/8(COG)
  Constant/1 -> Mux/1, Mux/2
  Update/1 -> Mux/3
  Mux/1 -> Product/2
  3vector LPF2/1(Out1) -> Sum6/1
  3vector LPF1/1(Out1) -> GyroBias/1, [bg_b], Scope/1
  Saturation/1 -> Embedded MATLAB Function1/2(pqr), Integer Delay5/1, Scope1/1

== system PositionComplementary4/Position/Attitude Filter/Enabled Subsystem ==
  In1 : Inport
  Enable : EnablePort
  Out1 : Outport
  wires:
  In1/1 -> Out1/1

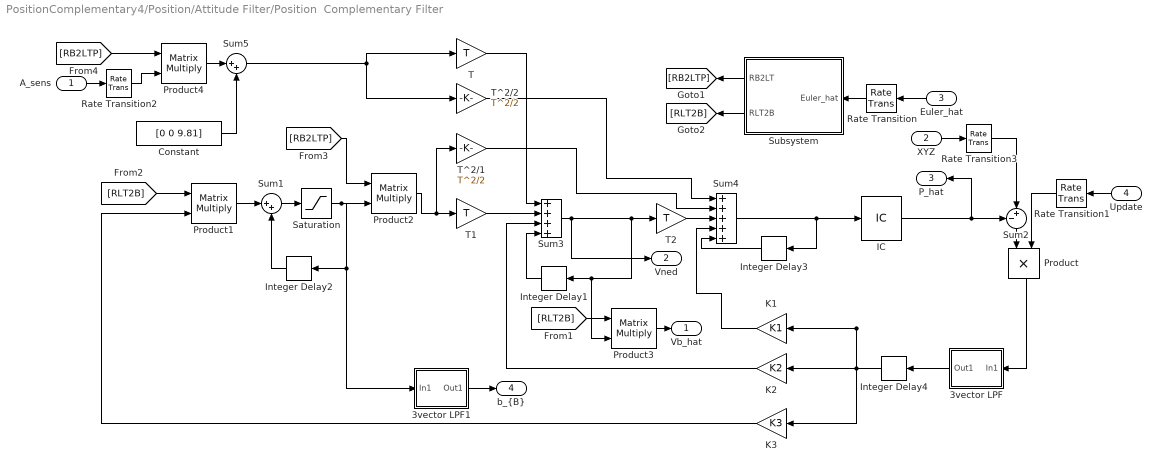
== system PositionComplementary4/Position/Attitude Filter/Position  Complementary Filter ==
  A_sens : Inport
  XYZ : Inport  Port=2
  Euler_hat : Inport  Orientation=left  Port=3
  Update : Inport  Orientation=left  Port=4
  3vector LPF : Subsystem  Orientation=left  mask{flpf=flpf, T=T}
      mask prompts: flpf "Low Pass Frequency (in S domain)"; T "Sample time"
      mask Display: droots([],-flpf,flpf)
  3vector LPF1 : Subsystem  mask{flpf=3, T=T}
      mask prompts: flpf "Low Pass Frequency (in S domain)"; T "Sample time"
      mask Display: droots([],-flpf,flpf)
  Constant : Constant  Value=[0 0 9.81]  SampleTime=0.01
  IC : InitialCondition  Value=P0  SampleTime=T
  Integer Delay{1..4} (4 alike) : simulink/Discrete/Integer Delay  Orientation=left  vinit=0.0  samptime=-1  NumDelays=1
  K1 : Gain  Orientation=left  Gain=K1
  K2 : Gain  Orientation=left  Gain=K2
  K3 : Gain  Orientation=left  Gain=K3
  Product : Product  Orientation=down  RndMeth=Zero
  Product{1..4} (4 alike) : Product  Multiplication=Matrix(*)  RndMeth=Zero
  Rate Transition : RateTransition  Orientation=left  OutPortSampleTime=T
  Rate Transition1 : RateTransition  Orientation=left  OutPortSampleTime=T
  Rate Transition2 : RateTransition  OutPortSampleTime=T
  Rate Transition3 : RateTransition  OutPortSampleTime=T
  Saturation : Saturate  UpperLimit=10  LowerLimit=-10
  Subsystem : Subsystem  Orientation=left
  Sum1 : Sum  Inputs=|++
  Sum2 : Sum  Orientation=down  Inputs=-+|
  Sum3 : Sum  Inputs=4
  Sum4 : Sum  Inputs=5
  Sum5 : Sum  Inputs=|++
  T : Gain  Gain=T
  T1 : Gain  Gain=T
  T2 : Gain  Gain=T
  T^2/1 : Gain  Gain=T^2/2
  T^2/2 : Gain  Gain=T^2/2
  Vb_hat : Outport
  Vned : Outport  Port=2
  P_hat : Outport  Orientation=left  Port=3
  "b_{B}" : Outport  Port=4
  wires:
  Subsystem/2(RLT2B) -> [RLT2B]
  Subsystem/1(RB2LT) -> [RB2LTP]
  Euler_hat/1 -> Rate Transition/1
  K3/1 -> Product1/2
  Product1/1 -> Sum1/1
  Sum1/1 -> Saturation/1
  Product2/1 -> T^2/1/1, T1/1
  T1/1 -> Sum3/2
  T/1 -> Sum3/1
  Sum3/1 -> T2/1, Integer Delay1/1, Product3/2, Vned/1
  K2/1 -> Sum3/3
  T2/1 -> Sum4/3
  T^2/1/1 -> Sum4/2
  T^2/2/1 -> Sum4/1
  Sum4/1 -> Integer Delay3/1, IC/1
  K1/1 -> Sum4/4
  XYZ/1 -> Rate Transition3/1
  Product3/1 -> Vb_hat/1
  Sum2/1 -> Product/1
  Product/1 -> 3vector LPF/1(In1)
  Update/1 -> Rate Transition1/1
  Integer Delay3/1 -> Sum4/5
  Integer Delay2/1 -> Sum1/2
  Integer Delay1/1 -> Sum3/4
  A_sens/1 -> Rate Transition2/1
  Product4/1 -> Sum5/1
  Constant/1 -> Sum5/2
  Sum5/1 -> T/1, T^2/2/1
  Rate Transition/1 -> Subsystem/1(Euler_hat)
  Rate Transition1/1 -> Product/2
  Rate Transition3/1 -> Sum2/2
  [RLT2B] -> Product1/1
  [RB2LTP] -> Product4/1
  Rate Transition2/1 -> Product4/2
  [RB2LTP] -> Product2/1
  [RLT2B] -> Product3/1
  IC/1 -> Sum2/1, P_hat/1
  Integer Delay4/1 -> K1/1, K2/1, K3/1
  3vector LPF/1(Out1) -> Integer Delay4/1
  3vector LPF1/1(Out1) -> "b_{B}"/1
  Saturation/1 -> Product2/2, Integer Delay2/1, 3vector LPF1/1(In1)

== system PositionComplementary4/Signal Cond/Accel Convert ==
  Raw : Inport
  3vector LPF : Subsystem  mask{flpf=5}
      mask prompts: flpf "LowPass Freq"
      mask Display: droots([],-flpf,flpf)
  Bias : Constant  Value=[2015 2018 2006]
  Divide : Product  Inputs=/*  OutScaling=2^-10
  Gains : Constant  Value=[-41 41 -43]
  Scope2 : Scope
      settings: TimeRange=100  YMin=-14.06123404388128  YMax=1.094597546893038  SaveName=ScopeData25
  Sum : Sum  Inputs=|+-
  Comp : Outport
  wires:
  Raw/1 -> 3vector LPF/1(In1)
  Divide/1 -> Comp/1, Scope2/1
  Sum/1 -> Divide/2
  Gains/1 -> Divide/1
  Bias/1 -> Sum/2
  3vector LPF/1(Out1) -> Sum/1

== system PositionComplementary4/Signal Cond/Gyro Convert ==
  Raw : Inport
  3vector LPF : Subsystem  mask{flpf=5}
      mask prompts: flpf "LowPass Freq"
      mask Display: droots([],-flpf,flpf)
  Bias : Constant  Value=[1866 1981 2042]
  Divide : Product  Inputs=/*  OutScaling=2^-10
  Gains : Constant  Value=[-142 142 235]
  Sum : Sum  Inputs=|+-
  Comp : Outport
  wires:
  Bias/1 -> Sum/2
  Gains/1 -> Divide/1
  Sum/1 -> Divide/2
  Divide/1 -> Comp/1
  Raw/1 -> 3vector LPF/1(In1)
  3vector LPF/1(Out1) -> Sum/1

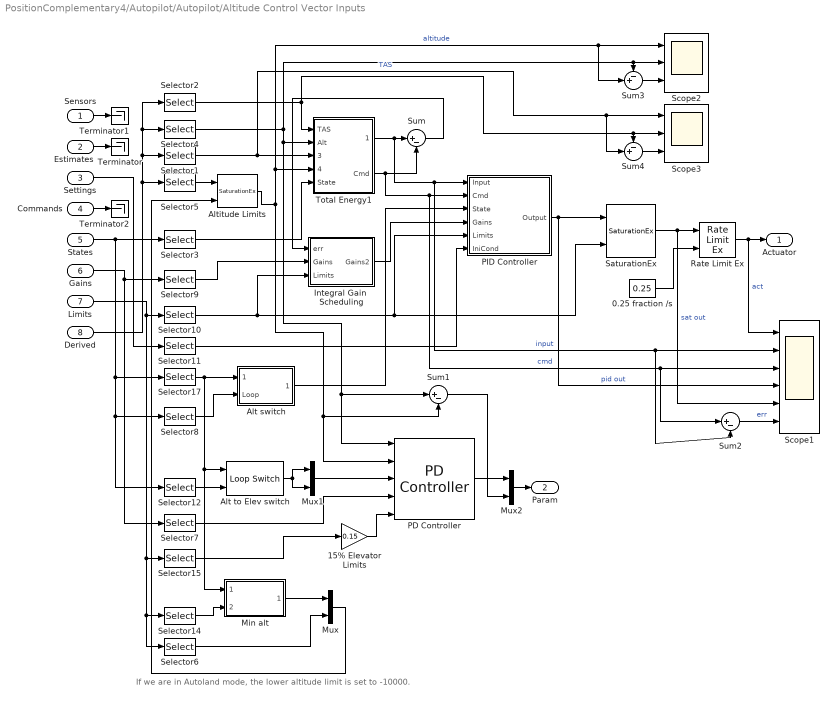
== system PositionComplementary4/Autopilot/Autopilot/Altitude Control Vector Inputs ==
  note: If we are in Autoland mode, the lower altitude limit is set to -10000.
  Sensors : Inport  PortDimensions=SizeSensors
  Estimates : Inport  Port=2  PortDimensions=SizeEstim
  Settings : Inport  Port=3  PortDimensions=SizeSet
  Commands : Inport  Port=4  PortDimensions=SizeCmd
  States : Inport  Port=5  PortDimensions=SizeStates
  Gains : Inport  Port=6  PortDimensions=SizeGains
  Limits : Inport  Port=7  PortDimensions=SizeLimits
  Derived : Inport  Port=8  PortDimensions=SizeDrv
  0.25 fraction /s : Constant  Value=0.25
  15% Elevator Limits : Gain  Gain=0.15  SaturateOnIntegerOverflow=on
  Alt switch : Subsystem  AncestorBlock=piccolo_library/Logic/DynP-Alt-Turn switch
  Alt to Elev switch : piccolo_library/Logic/Loop Switch  SystemSampleTime=-1
  Altitude Limits : piccolo_library/Nonlinear/SaturationEx  SystemSampleTime=-1
  Integral Gain  Scheduling : Subsystem
  Min alt : Subsystem
      mask Type: Loop Switch
      mask Description:
      | Select whether this individual loop is enabled or disabled.  This is done based on the specific
      | loop enable state, and the global flag.  In auto or manual steering the loop is on.  In Manual
      | or AutoLaunch the loop should be off.
  Mux : Mux  Inputs=2
  Mux1 : Mux  Inputs=2
  Mux2 : Mux  Inputs=2
  PD Controller : piccolo_library/Controllers/PD Controller  SystemSampleTime=-1  tsamp=tsamp  tdelay=0.5
  PID Controller : Subsystem  AncestorBlock=piccolo_library/Controllers/PID Controller  mask(PID Controller){tsamp=tsamp, tdelay=1}
      mask prompts: tsamp "Sample time:"; tdelay "Time derivative delay:"
      mask help: Generic PID (proportional, integral, derivative) controller with a single input and a single output.
  Rate Limit Ex : piccolo_library/Nonlinear/Rate Limit Ex  SystemSampleTime=-1  T=tsamp
  SaturationEx : piccolo_library/Nonlinear/SaturationEx  SystemSampleTime=-1
  Scope1 : Scope  NumInputPorts=6
      settings: YMin=0.120001~972.462~972.462~0.120001~0.120001~5.25e-006  YMax=0.120001~972.462~972.462~0.120001~0.120001~7e-006
  Scope2 : Scope  NumInputPorts=3
      settings: YMin=855~900.05~-0.475  YMax=945~900.475~-0.05  SaveName=ScopeData14
  Scope3 : Scope  NumInputPorts=3
      settings: YMin=35.0006~35~-0.035  YMax=35.0008~35.035~3.46945e-018  SaveName=ScopeData17
  Selector1 : Selector  IndexOptions=Index vector (dialog)  Indices=IdxDrvTASCmdNom  OutputSizes=1  InputPortWidth=SizeDrv
  Selector10 : Selector  IndexOptions=Index vector (dialog)  Indices=[IdxLimitsThrottleMin IdxLimitsThrottleMax]  OutputSizes=1  InputPortWidth=SizeLimits
  Selector11 : Selector  IndexOptions=Index vector (dialog)  Indices=IdxSetThrottleTrim  OutputSizes=1  InputPortWidth=SizeSet
  Selector12 : Selector  IndexOptions=Index vector (dialog)  Indices=IdxStatesAltToElev  OutputSizes=1  InputPortWidth=SizeStates
  Selector14 : Selector  IndexOptions=Index vector (dialog)  Indices=IdxLimitsAltMin  OutputSizes=1  InputPortWidth=SizeLimits
  Selector15 : Selector  IndexOptions=Index vector (dialog)  Indices=[IdxLimitsElevatorMin IdxLimitsElevatorMax]  OutputSizes=1  InputPortWidth=SizeLimits
  Selector17 : Selector  IndexOptions=Index vector (dialog)  Indices=[IdxStatesGlobal IdxStatesMode IdxStatesManual]  OutputSizes=1  InputPortWidth=SizeStates
  Selector2 : Selector  IndexOptions=Index vector (dialog)  Indices=IdxDrvTAS  OutputSizes=1  InputPortWidth=SizeDrv
  Selector3 : Selector  IndexOptions=Index vector (dialog)  Indices=IdxStatesPdyn  OutputSizes=1  InputPortWidth=SizeStates
  Selector4 : Selector  IndexOptions=Index vector (dialog)  Indices=IdxDrvBaroAlt  OutputSizes=1  InputPortWidth=SizeDrv
  Selector5 : Selector  IndexOptions=Index vector (dialog)  Indices=IdxDrvAltCmd  OutputSizes=1  InputPortWidth=SizeDrv
  Selector6 : Selector  IndexOptions=Index vector (dialog)  Indices=IdxLimitsAltMax  OutputSizes=1  InputPortWidth=SizeLimits
  Selector7 : Selector  IndexOptions=Index vector (dialog)  Indices=[IdxGainsSlopeElevatorP IdxGainsSlopeElevatorD]  OutputSizes=1  InputPortWidth=SizeGains
  Selector8 : Selector  IndexOptions=Index vector (dialog)  Indices=IdxStatesAlt  OutputSizes=1  InputPortWidth=SizeStates
  Selector9 : Selector  IndexOptions=Index vector (dialog)  Indices=[IdxGainsAltP IdxGainsAltI IdxGainsAltD]  OutputSizes=1  InputPortWidth=SizeGains
  Sum : Sum  Inputs=|+-  SaturateOnIntegerOverflow=on
  Sum1 : Sum  Inputs=|+-  SaturateOnIntegerOverflow=on
  Sum2 : Sum  Inputs=|+-  SaturateOnIntegerOverflow=on
  Sum3 : Sum  Inputs=-+|  SaturateOnIntegerOverflow=on
  Sum4 : Sum  Inputs=-+|  SaturateOnIntegerOverflow=on
  Terminator : Terminator
  Terminator1 : Terminator
  Terminator2 : Terminator
  Total Energy1 : Subsystem
      mask Type: Total Energy
      mask Description: Compute the total energy state and command as a sum of kinetic and potential energies, in units of altitude
  Actuator : Outport  OutDataType=fixdt(1,16,0)  OutScaling=[]
  Param : Outport  Port=2  OutDataType=fixdt(1,16,0)  OutScaling=[]
  wires:
  Total Energy1/2(Cmd) -> Sum/2, PID Controller/2(Cmd), Scope1/3, Sum2/1  "cmd"
  Total Energy1/1(Energy) -> Sum/1, PID Controller/1(Input), Scope1/2, Sum2/2  "input"
  Selector3/1 -> Total Energy1/5(State)
  Selector1/1 -> Total Energy1/3(TASCmd), Scope3/1, Sum4/2  "TAS"
  PD Controller/1 -> Mux2/1
  Mux2/1 -> Param/1
  Sum1/1 -> Mux2/2
  Commands/1 -> Terminator2/1
  States/1 -> Selector3/1, Selector12/1, Selector8/1, Selector17/1
  Sum/1 -> Integral Gain  Scheduling/1(err)
  Selector7/1 -> PD Controller/4
  Mux1/1 -> PD Controller/3
  Alt to Elev switch/1 -> Mux1/2, Mux1/1
  Selector15/1 -> 15% Elevator Limits/1
  15% Elevator Limits/1 -> PD Controller/5
  Selector9/1 -> Integral Gain  Scheduling/2(Gains)
  Integral Gain  Scheduling/1(Gains2) -> PID Controller/4(Gains)
  Mux/1 -> Altitude Limits/2
  Selector6/1 -> Mux/2
  Min alt/1(MinAltOut) -> Mux/1
  Selector14/1 -> Min alt/2(MinAlt)
  Selector12/1 -> Alt to Elev switch/2
  PID Controller/1(Output) -> SaturationEx/1, Scope1/4  "pid out"
  Derived/1 -> Selector1/1, Selector4/1, Selector2/1, Selector5/1
  Selector5/1 -> Altitude Limits/1
  Altitude Limits/1 -> Sum1/2, PD Controller/2, Total Energy1/4(AltCmd), Scope2/1, Sum3/2  "altitude"
  Selector4/1 -> Total Energy1/2(Alt), Sum1/1, PD Controller/1, Scope2/2, Sum3/1
  Selector2/1 -> Total Energy1/1(TAS), Scope3/2, Sum4/1
  Sensors/1 -> Terminator1/1
  Rate Limit Ex/1 -> Actuator/1, Scope1/1  "act"
  0.25 fraction /s/1 -> Rate Limit Ex/2
  SaturationEx/1 -> Rate Limit Ex/1, Scope1/5  "sat out"
  Selector10/1 -> Integral Gain  Scheduling/3(Limits), SaturationEx/2, PID Controller/5(Limits)
  Limits/1 -> Selector15/1, Selector6/1, Selector14/1, Selector10/1
  Gains/1 -> Selector7/1, Selector9/1
  Selector11/1 -> PID Controller/6(IniCond)
  Settings/1 -> Selector11/1
  Selector17/1 -> Alt switch/1(Globals), Min alt/1(Globals), Alt to Elev switch/1
  Selector8/1 -> Alt switch/2(Loop)
  Alt switch/1(TriOut) -> PID Controller/3(State)
  Estimates/1 -> Terminator/1
  Sum2/1 -> Scope1/6  "err"
  Sum3/1 -> Scope2/3
  Sum4/1 -> Scope3/3

== system PositionComplementary4/Autopilot/Autopilot/Flap Control Vector Inputs ==
  Sensors : Inport  PortDimensions=SizeSensors
  Estimates : Inport  Port=2  PortDimensions=SizeEstim
  Settings : Inport  Port=3  PortDimensions=SizeSet
  Commands : Inport  Port=4  PortDimensions=SizeCmd
  States : Inport  Port=5  PortDimensions=SizeStates
  Gains : Inport  Port=6  PortDimensions=SizeGains
  Limits : Inport  Port=7  PortDimensions=SizeLimits
  Derived : Inport  Port=8  PortDimensions=SizeDrv
  5 deg/s : Constant  Value=10*pi/180
  Direct Flap Control : Selector  IndexOptions=Index vector (dialog)  Indices=IdxCmdFlap  OutputSizes=1  InputPortWidth=SizeCmd
  Flap Loop Switch : piccolo_library/Logic/Loop Switch  SystemSampleTime=-1
  Landing Flap : Selector  IndexOptions=Index vector (dialog)  Indices=IdxSetLandingFlap  OutputSizes=1  InputPortWidth=SizeSet
  Rate Limit Ex : piccolo_library/Nonlinear/Rate Limit Ex  SystemSampleTime=-1  T=tsamp
  SaturationEx : piccolo_library/Nonlinear/SaturationEx  SystemSampleTime=-1
  Selector1 : Selector  IndexOptions=Index vector (dialog)  Indices=[IdxStatesGlobal IdxStatesMode IdxStatesManual]  OutputSizes=1  InputPortWidth=SizeStates
  Selector10 : Selector  IndexOptions=Index vector (dialog)  Indices=[IdxLimitsFlapMin IdxLimitsFlapMax]  OutputSizes=1  InputPortWidth=SizeLimits
  Selector12 : Selector  IndexOptions=Index vector (dialog)  Indices=IdxStatesSlope  OutputSizes=1  InputPortWidth=SizeStates
  Selector2 : Selector  IndexOptions=Index vector (dialog)  Indices=IdxStatesFlap  OutputSizes=1  InputPortWidth=SizeStates
  Switch : Switch  Threshold=0.5  SaturateOnIntegerOverflow=on
  Switch1 : Switch  Threshold=0.5  SaturateOnIntegerOverflow=on
  Terminator{1..4} (4 alike) : Terminator
  Zero : Constant  Value=0
  Actuator : Outport  OutDataType=fixdt(1,16,0)  OutScaling=[]
  wires:
  Sensors/1 -> Terminator1/1
  Selector10/1 -> SaturationEx/2
  Selector12/1 -> Switch/2
  Direct Flap Control/1 -> Switch/3
  Landing Flap/1 -> Switch/1
  Estimates/1 -> Terminator2/1
  Gains/1 -> Terminator3/1
  Derived/1 -> Terminator4/1
  Settings/1 -> Landing Flap/1
  Commands/1 -> Direct Flap Control/1
  States/1 -> Selector12/1, Selector2/1, Selector1/1
  Limits/1 -> Selector10/1
  Switch/1 -> Switch1/1
  Flap Loop Switch/1 -> Switch1/2
  Switch1/1 -> SaturationEx/1
  Selector1/1 -> Flap Loop Switch/1
  Selector2/1 -> Flap Loop Switch/2
  Zero/1 -> Switch1/3
  SaturationEx/1 -> Rate Limit Ex/1
  Rate Limit Ex/1 -> Actuator/1
  5 deg/s/1 -> Rate Limit Ex/2
